simulink model "bh_test_virtual_camera_model"  (R2017b)
settings: Solver=ode45  StartTime=0.0  StopTime=15  RelTol=1e-5  EnableMultiTasking=on
undefined symbols (not defined in the file or in its folder): gray
libraries: visiongeotforms x1, bh_cv_car_drc_library x1
settings Model: Creator=sriramn  LastModifiedBy=bhorton
settings SolverCC: ZeroCrossAlgorithm=Adaptive
settings DataIOCC: LimitDataPoints=on  SaveFormat=Array
settings OptimizationCC: LifeSpan=inf
settings DebuggingCC: AlgebraicLoopMsg=error  SolverPrmCheckMsg=warning  AllowSymbolicDim=off  SFUnexpectedBacktrackingDiag=warning  SFNoUnconditionalDefaultTransitionDiag=warning  SFExecutionAtInitializationDiag=none
settings HardwareCC: ProdBitPerPointer=32  ProdBitPerSizeT=32  ProdBitPerPtrDiffT=32  ProdLargestAtomicFloat=None  ProdIntDivRoundTo=Undefined  ProdEndianess=Unspecified  ProdWordSize=32  ProdHWDeviceType=32-bit Generic
settings ModelReferenceCC: PropagateSignalLabelsOutOfModel=off
settings CodeAppCC: StateflowObjectComments=on
settings GRTTargetCC: TargetLangStandard=C89/C90 (ANSI)  GeneratePreprocessorConditionals=Disable all
settings ConfigComp: CovMetricSettings=dw  CovHtmlReporting=on  CovSaveCumulativeToWorkspaceVar=on  CovSaveSingleToWorkspaceVar=on  CovExternalEMLEnable=off  CovSFcnEnable=off
settings SimscapeCC: SimscapeNormalizeSystem=off
settings ConfigurationSet: Description=SimMechanics 2G
settings ExplorerConfigSet: InternalSimMechanicsExplorerSettings="<ExplorerConfiguration><canonicalview>planar_xy</canonicalview><AnimationSetting><BasePlaybackSpeed>1.0</BasePlaybackSpeed><PlaybackSpeedFactor>1.0</PlaybackSpeedFactor></AnimationSetting><TilePanel><TileInfo><Tiles Columns=\"1\" Count=\"1\" Rows=\"1\"><Column Left=\"2\" Weight=\"1\"/><Column Left=\"1628\"/><Row Top=\"2\" Weight=\"1\"/><Row Top=\"1072\"/><Tile Height=\"1\" Width=\"1\" X=\"0\" Y=\"0\"/></Tiles></TileInfo><SceneInfo><SceneViewer><BGColor><R>0.60000002384185791</R><G>0.60000002384185791</G><B>0.60000002384185791</B></BGColor><Camera><Position><X>0.22951840878551699</X><Y>0.32651610611526627</Y><Z>-0.27215421354393321</Z></Position><Center><X>-0.15775714411666431</X><Y>-0.15462825985839526</Y><Z>0.065702552916005602</Z></Center><Up><X>-0.56030137557930915</X><Y>0.72817587161684794</Y><Z>0.39474329445726858</Z></Up><Left>-0.21481383955700509</Left><Right>0.21481383955700509</Right><Bottom>-0.27569784609469139</Bottom><Top>0.27569784609469139</Top></Camera></SceneViewer></SceneInfo></TilePanel></ExplorerConfiguration>"

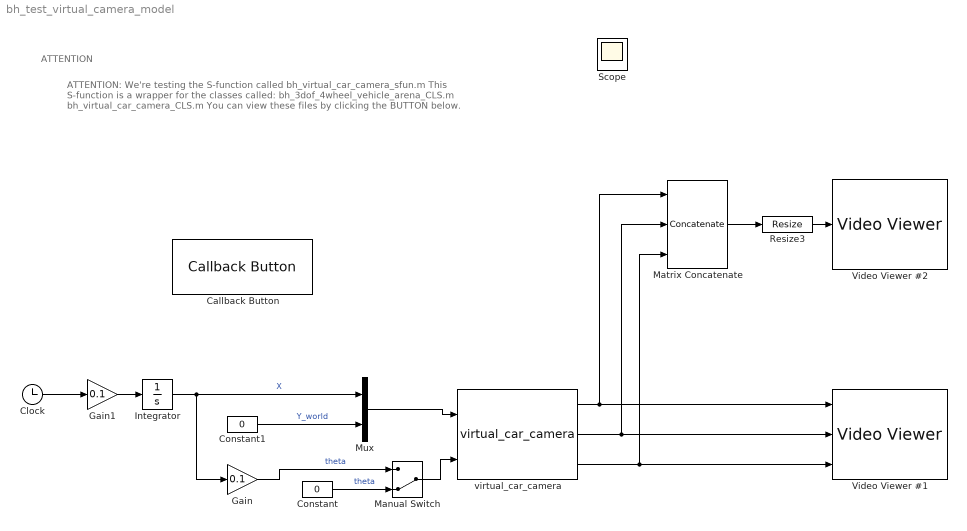
== system bh_test_virtual_camera_model ==
  note: ATTENTION
  note: ATTENTION:
      |
      | We're testing the S-function called bh_virtual_car_camera_sfun.m
      |
      | This S-function is a wrapper for the classes called:
      | bh_3dof_4wheel_vehicle_arena_CLS.m
      | bh_virtual_car_camera_CLS.m
      |
      | You can view these files by clicking the BUTTON below.
  Callback Button : CallbackButton  WebBlockId=5640  ButtonText=View M-files  PressDelay=500  RepeatInterval=0
      settings: ClickFcn=|
      | edit('bh_virtual_car_camera_sfun.m', ...
      |      'bh_3dof_4wheel_vehicle_arena_CLS.m', ...
      |      'bh_virtual_car_camera_CLS.m')
  Clock : Clock
  Constant : Constant  Value=0
  Constant1 : Constant  Value=0
  Gain : Gain  Gain=0.1
  Gain1 : Gain  Gain=0.1
  Integrator : Integrator
  Manual Switch : ManualSwitch  CurrentSetting=0
  Matrix Concatenate : Concatenate  NumInputs=3  Mode=Multidimensional array  ConcatenateDimension=3
  Mux : Mux  Inputs=2
  Resize3 : visiongeotforms/Resize  specify=Number of output rows and columns  rfactor=[200 150]  outCols=25  outRows=25  outRowsCols=[120 160]  interp_method=Bilinear  antialias=on  useROI=off  roiFlag=off  prodOutputMode=Binary point scaling  prodOutputWordLength=32  prodOutputFracLength=10  roundingMode=Nearest  overflowMode=on
      settings: SourceProductName=Computer Vision System Toolbox  SourceProductBaseCode=VP
  Video Viewer #1 : VideoViewer  imagePorts=separate color signals  FigPos=[1261 430 418 304]
  Video Viewer #2 : VideoViewer  colormapValue=gray(256)  FigPos=[1293 946 418 304]
  virtual_car_camera : bh_cv_car_drc_library/CAR_things/virtual_car_camera  obstacle_visibility=SHOW_OBSTACLES  W=320  H=240  Ts=0.1  init_cam_pos_wrt_W=[0,0]  height_of_cam=0.4  init_veh_THETA_wrt_W=0  horz_look_dist=100  cam_va=11
  Scope : Scope
  wires:
  Integrator/1 -> Gain/1, Mux/1  "X"
  Constant1/1 -> Mux/2  "Y_world"
  Mux/1 -> virtual_car_camera/1
  Clock/1 -> Gain1/1
  virtual_car_camera/1 -> Matrix Concatenate/1, Video Viewer #1/1
  virtual_car_camera/2 -> Matrix Concatenate/2, Video Viewer #1/2
  virtual_car_camera/3 -> Matrix Concatenate/3, Video Viewer #1/3
  Constant/1 -> Manual Switch/2  "theta"
  Manual Switch/1 -> virtual_car_camera/2
  Gain/1 -> Manual Switch/1  "theta"
  Gain1/1 -> Integrator/1
  Resize3/1 -> Video Viewer #2/1
  Matrix Concatenate/1 -> Resize3/1
